simulink subsystem "Gyroscope"  (R2024b)
settings: Solver=VariableStepAuto  StartTime=0.0  StopTime=10.0  RelTol=1e-3
values from neighbouring files (symbols this model uses):
  Ts = 1e-2    (= 0.01)    [Plant_balrob_params.m]
settings Model: Creator=federico  LastModifiedBy=federico

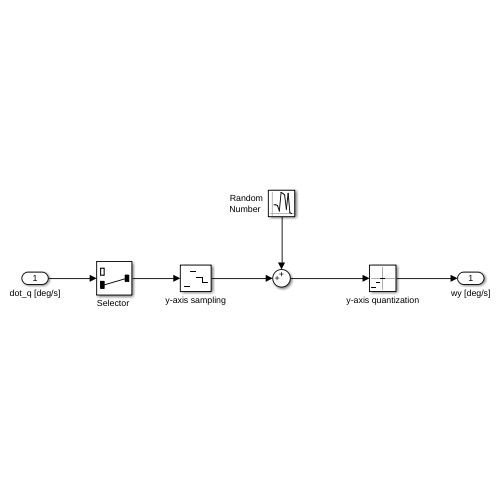
[thumbnail: Simulink's stored preview of the top-level diagram]
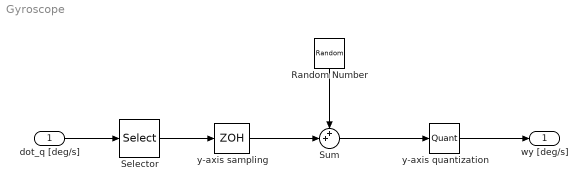
== system Gyroscope ==
  dot_q [deg/s] : Inport
  "Random Number " : RandomNumber  Variance=sens.mpu.gyro.noisevar  SampleTime=Ts
  "Selector " : Selector  InputPortWidth=2  IndexOptions=Index vector (dialog)  Indices=[2]  OutputSizes=1
  Sum : Sum  Inputs=++|
  y-axis quantization : Quantizer  QuantizationInterval=sens.mpu.gyro.LSB2degs
  y-axis sampling : ZeroOrderHold  SampleTime=Ts
  wy [deg/s] : Outport
  wires:
  dot_q [deg/s]/1 -> "Selector "/1
  "Selector "/1 -> y-axis sampling/1
  y-axis sampling/1 -> Sum/2
  "Random Number "/1 -> Sum/1
  Sum/1 -> y-axis quantization/1
  y-axis quantization/1 -> wy [deg/s]/1
